simulink model "MedicalRoboticsProject"  (Simulink 8.5)
settings: Solver=ode4  StartTime=0.0  StopTime=20  FixedStep=0.01  RelTol=1e-3
model workspace (MAT data in the model file):
  Kx = 5
  Ky = 1.5
  Kz = 2
  x = 3
  y = 3
  z = 3
  K1 = 1
  K2 = 1
  K3 = 1
  K4 = 1
  K5 = 1
  K6 = 1
  Fx = 1
  Fy = 1
  Fz = 0.5
  F1 = 0
  F2 = -0.5
  F3 = 0
  xg = 4
  yg = 4
  zg : num (value not decoded)
values from neighbouring files (symbols this model uses):
  z = T(1:3,1:3)*z0    [DH.m]
settings Model: Creator=ahmad  LastModifiedBy=ahmad
settings DataIOCC: SignalLoggingSaveFormat=Dataset
settings OptimizationCC: ExpressionDepthLimit=128
settings DebuggingCC: UnderspecifiedInitializationDetection=Simplified  MergeDetectMultiDrivingBlocksExec=error  FcnCallInpInsideContextMsg=EnableAllAsError  StateNameClashWarn=none
settings GRTTargetCC: CombineOutputUpdateFcns=on  GRTInterface=off

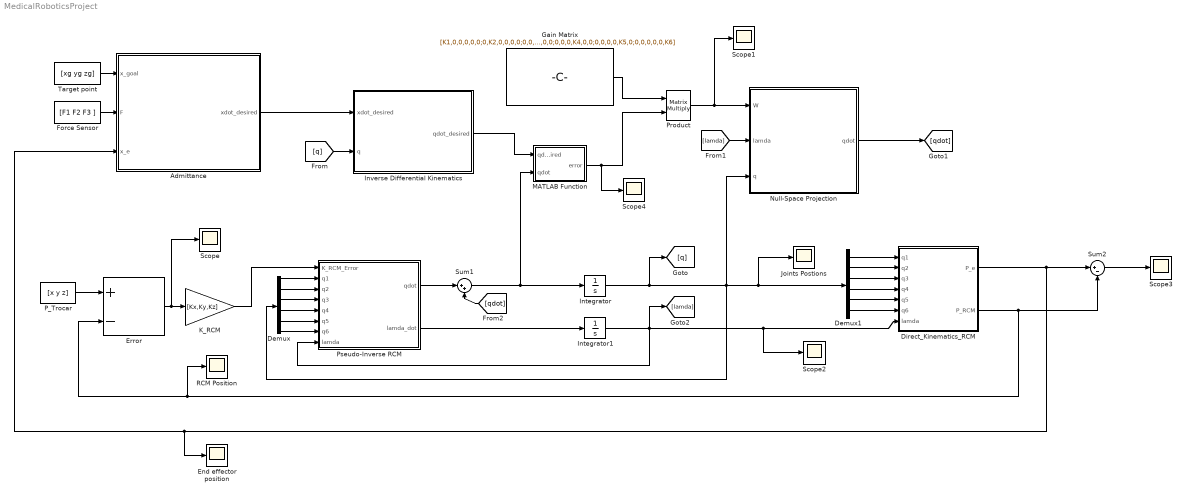
== system MedicalRoboticsProject ==
  Admittance : MATLAB Function  TreatAsAtomicUnit=on
  Demux : Demux  Outputs=6
  Demux1 : Demux  Outputs=6
  Direct_Kinematics_RCM : MATLAB Function  TreatAsAtomicUnit=on
  End effector position : Scope
      settings: YMin=-5e-12  YMax=2.5e-11  SaveName=ScopeData3
  Error : Sum  Inputs=+-
  Force Sensor : Constant  Value=[F1 F2 F3 ]
  Gain Matrix : Constant  Value=[K1,0,0,0,0,0;0,K2,0,0,0,0;0,0,K3,0,0,0;0,0,0,K4,0,0;0,0,0,0,K5,0;0,0,0,0,0,K6]  VectorParams1D=off
  Integrator : Integrator  InitialCondition=[1 1 1 pi/4 pi/4 1]
  Integrator1 : Integrator  InitialCondition=1  LimitOutput=on  UpperSaturationLimit=1  LowerSaturationLimit=0
  "Inverse Differential Kinematics " : MATLAB Function  TreatAsAtomicUnit=on
  Joints Postions : Scope
      settings: SaveName=ScopeData2
  K_RCM : Gain  Gain=[Kx,Ky,Kz]
  MATLAB Function : MATLAB Function  TreatAsAtomicUnit=on
  Null-Space Projection : MATLAB Function  TreatAsAtomicUnit=on
  P_Trocar : Constant  Value=[x y z]
  Product : Product  Multiplication=Matrix(*)
  "Pseudo-Inverse RCM " : MATLAB Function  TreatAsAtomicUnit=on
  RCM Position : Scope
      settings: YMin=-5e-12  YMax=2.5e-11  SaveName=ScopeData5
  Scope{,1..4} (5 alike) : Scope
      Scope settings: YMin=-5e-12  YMax=2.5e-11
      Scope2 settings: SaveName=ScopeData4
      Scope3 settings: SaveName=ScopeData6
      Scope4 settings: SaveName=ScopeData7
  Sum1 : Sum  Inputs=|++
  Sum2 : Sum  Inputs=|+-
  Target point : Constant  Value=[xg yg zg]
  wires:
  Demux/1 -> "Pseudo-Inverse RCM "/2(q1)
  Demux/2 -> "Pseudo-Inverse RCM "/3(q2)
  Demux/3 -> "Pseudo-Inverse RCM "/4(q3)
  Demux/4 -> "Pseudo-Inverse RCM "/5(q4)
  Demux/5 -> "Pseudo-Inverse RCM "/6(q5)
  Demux/6 -> "Pseudo-Inverse RCM "/7(q6)
  "Pseudo-Inverse RCM "/2(lamda_dot) -> Integrator1/1
  Integrator1/1 -> Scope2/1, Direct_Kinematics_RCM/7(lamda), [lamda], "Pseudo-Inverse RCM "/8(lamda)
  Integrator/1 -> [q], Null-Space Projection/3(q), Demux/1, Joints Postions/1, Demux1/1
  Demux1/1 -> Direct_Kinematics_RCM/1(q1)
  Demux1/2 -> Direct_Kinematics_RCM/2(q2)
  Demux1/3 -> Direct_Kinematics_RCM/3(q3)
  Demux1/4 -> Direct_Kinematics_RCM/4(q4)
  Demux1/5 -> Direct_Kinematics_RCM/5(q5)
  Demux1/6 -> Direct_Kinematics_RCM/6(q6)
  P_Trocar/1 -> Error/1
  Direct_Kinematics_RCM/2(P_RCM) -> RCM Position/1, Error/2, Sum2/2
  Error/1 -> Scope/1, K_RCM/1
  Target point/1 -> Admittance/1(x_goal)
  Force Sensor/1 -> Admittance/2(F)
  Admittance/1(xdot_desired) -> "Inverse Differential Kinematics "/1(xdot_desired)
  "Inverse Differential Kinematics "/1(qdot_desired) -> MATLAB Function/1(qdot_desired)
  "Pseudo-Inverse RCM "/1(qdot) -> Sum1/1
  [q] -> "Inverse Differential Kinematics "/2(q)
  [lamda] -> Null-Space Projection/2(lamda)
  Gain Matrix/1 -> Product/1
  Product/1 -> Null-Space Projection/1(W), Scope1/1
  Null-Space Projection/1(qdot) -> [qdot]
  K_RCM/1 -> "Pseudo-Inverse RCM "/1(K_RCM_Error)
  Sum1/1 -> Integrator/1, MATLAB Function/2(qdot)
  MATLAB Function/1(error) -> Scope4/1, Product/2
  Direct_Kinematics_RCM/1(P_e) -> Sum2/1, Admittance/3(x_e), End effector position/1
  [qdot] -> Sum1/2
  Sum2/1 -> Scope3/1

== matlab function Direct_Kinematics_RCM ==
  data: P_e output double; q1 input double; P_RCM output double; q2 input double; q3 input double; q4 input double; q5 input double; q6 input double; lamda input double
function [P_e, P_RCM]= fcn(q1, q2, q3, q4, q5, q6, lamda)
%#codegen
%p5 = [q2 + 5*sin(q4); q3 - (5*cos(q4)*(2^(1/2) + 2)^(1/2))/2 - 5*(2 - 2^(1/2))^(1/2); q1 + 5*(2^(1/2) + 2)^(1/2) - (5*cos(q4)*(2 - 2^(1/2))^(1/2))/2];
%p6 = [q2 + 5*sin(q4) - q6*cos(q4)*sin(q5); q3 - q6*((cos(q5)*(2 - 2^(1/2))^(1/2))/2 + (sin(q4)*sin(q5)*(2^(1/2) + 2)^(1/2))/2) - (5*cos(q4)*(2^(1/2) + 2)^(1/2))/2 - 5*(2 - 2^(1/2))^(1/2); q1 + 5*(2^(1/2) + 2)^(1/2) + q6*((cos(q5)*(2^(1/2) + 2)^(1/2))/2 - (sin(q4)*sin(q5)*(2 - 2^(1/2))^(1/2))/2) - (5*cos(q4)*(2 - 2^(1/2))^(1/2))/2];

p5 = [q2 + 5*cos(q4)*cos(q5)
      q3 - 5*(2 - 2^(1/2))^(1/2) - (5*sin(q5)*(2 - 2^(1/2))^(1/2))/2 + (5*cos(q5)*sin(q4)*(2^(1/2) + 2)^(1/2))/2
      q1 + 5*(2^(1/2) + 2)^(1/2) + (5*sin(q5)*(2^(1/2) + 2)^(1/2))/2 + (5*cos(q5)*sin(q4)*(2 - 2^(1/2))^(1/2))/2];
 

p6 =  [q2 + 5*cos(q4)*cos(q5) - q6*cos(q4)*sin(q5)
       q3 - q6*((cos(q5)*(2 - 2^(1/2))^(1/2))/2 + (sin(q4)*sin(q5)*(2^(1/2) + 2)^(1/2))/2) - 5*(2 - 2^(1/2))^(1/2) - (5*sin(q5)*(2 - 2^(1/2))^(1/2))/2 + (5*cos(q5)*sin(q4)*(2^(1/2) + 2)^(1/2))/2
       q1 + 5*(2^(1/2) + 2)^(1/2) + q6*((cos(q5)*(2^(1/2) + 2)^(1/2))/2 - (sin(q4)*sin(q5)*(2 - 2^(1/2))^(1/2))/2) + (5*sin(q5)*(2^(1/2) + 2)^(1/2))/2 + (5*cos(q5)*sin(q4)*(2 - 2^(1/2))^(1/2))/2];
 
P_RCM = p5 + lamda*(p6-p5);
P_e = p6;

== matlab function Pseudo-Inverse RCM  ==
  data: K_RCM_Error input double; q1 input double; q2 input double; q3 input double; q4 input double; qdot output double; q5 input double; q6 input double; lamda input double; lamda_dot output double
function [qdot,lamda_dot] = fcn(K_RCM_Error, q1, q2, q3, q4, q5, q6, lamda)
%#codegen
%coder.extrinsic('simplify'); 

% Jl1 = [0;0;1];
% Jl2 = [1;0;0];
% Jl3 = [0;1;0];
% Jl4 = [5*cos(q4) + q6*sin(q4)*sin(q5); ((5*sin(q4) - q6*cos(q4)*sin(q5))*(2^(1/2) + 2)^(1/2))/2; ((5*sin(q4) - q6*cos(q4)*sin(q5))*(2 - 2^(1/2))^(1/2))/2];

% Jl4 = simplify(Jl4);
% Jl5 = [-q6*cos(q4)*cos(q5); q6*((sin(q5)*(2 - 2^(1/2))^(1/2))/2 - (cos(q5)*sin(q4)*(2^(1/2) + 2)^(1/2))/2); -q6*((sin(q5)*(2^(1/2) + 2)^(1/2))/2 + (cos(q5)*sin(q4)*(2 - 2^(1/2))^(1/2))/2)];
% Jl5 = simplify(Jl5);
% Jl6 = [-cos(q4)*sin(q5);-(cos(q5)*(2 - 2^(1/2))^(1/2))/2 - (sin(q4)*sin(q5)*(2^(1/2) + 2)^(1/2))/2; (cos(q5)*(2^(1/2) + 2)^(1/2))/2 - (sin(q4)*sin(q5)*(2 - 2^(1/2))^(1/2))/2];
% Jl6 =  simplify(Jl6);


%J_5 = [0,1,0,5*cos(q4) + q6*sin(q4)*sin(q5),-q6*cos(q4)*cos(q5),0; 0,0,1,((5*sin(q4) - q6*cos(q4)*sin(q5))*(2^(1/2) + 2)^(1/2))/2,q6*((sin(q5)*(2 - 2^(1/2))^(1/2))/2 - (cos(q5)*sin(q4)*(2^(1/2) + 2)^(1/2))/2),0; 1,0,0,((5*sin(q4) - q6*cos(q4)*sin(q5))*(2 - 2^(1/2))^(1/2))/2,-q6*((sin(q5)*(2^(1/2) + 2)^(1/2))/2 + (cos(q5)*sin(q4)*(2 - 2^(1/2))^(1/2))/2),0];
% J_5 = [Jl1,Jl2,Jl3,Jl4,Jl5,0;0;0];
%J_6 = [Jl1,Jl2,Jl3,Jl4,Jl5,Jl6];
%J_6 = [0,1,0,5*cos(q4) + q6*sin(q4)*sin(q5),-q6*cos(q4)*cos(q5),-cos(q4)*sin(q5); 0,0,1,((5*sin(q4) - q6*cos(q4)*sin(q5))*(2^(1/2) + 2)^(1/2))/2,q6*((sin(q5)*(2 - 2^(1/2))^(1/2))/2 - (cos(q5)*sin(q4)*(2^(1/2) + 2)^(1/2))/2),-(cos(q5)*(2 - 2^(1/2))^(1/2))/2 - (sin(q4)*sin(q5)*(2^(1/2) + 2)^(1/2))/2; 1,0,0,((5*sin(q4) - q6*cos(q4)*sin(q5))*(2 - 2^(1/2))^(1/2))/2,-q6*((sin(q5)*(2^(1/2) + 2)^(1/2))/2 + (cos(q5)*sin(q4)*(2 - 2^(1/2))^(1/2))/2),(cos(q5)*(2^(1/2) + 2)^(1/2))/2 - (sin(q4)*sin(q5)*(2 - 2^(1/2))^(1/2))/2];

J_5 = [0, 1, 0, -sin(q4)*(5*cos(q5) - q6*sin(q5)), -cos(q4)*(5*sin(q5) + q6*cos(q5)), 0
       0, 0, 1, (cos(q4)*(5*cos(q5) - q6*sin(q5))*(2^(1/2) + 2)^(1/2))/2, q6*((sin(q5)*(2 - 2^(1/2))^(1/2))/2 - (cos(q5)*sin(q4)*(2^(1/2) + 2)^(1/2))/2) - (5*cos(q5)*(2 - 2^(1/2))^(1/2))/2 - (5*sin(q4)*sin(q5)*(2^(1/2) + 2)^(1/2))/2, 0
       1, 0, 0, (cos(q4)*(5*cos(q5) - q6*sin(q5))*(2 - 2^(1/2))^(1/2))/2, (5*cos(q5)*(2^(1/2) + 2)^(1/2))/2 - q6*((sin(q5)*(2^(1/2) + 2)^(1/2))/2 + (cos(q5)*sin(q4)*(2 - 2^(1/2))^(1/2))/2) - (5*sin(q4)*sin(q5)*(2 - 2^(1/2))^(1/2))/2, 0];

J_6 = [0, 1, 0, -sin(q4)*(5*cos(q5) - q6*sin(q5)), -cos(q4)*(5*sin(q5) + q6*cos(q5)), -cos(q4)*sin(q5)
       0, 0, 1, (cos(q4)*(5*cos(q5) - q6*sin(q5))*(2^(1/2) + 2)^(1/2))/2, q6*((sin(q5)*(2 - 2^(1/2))^(1/2))/2 - (cos(q5)*sin(q4)*(2^(1/2) + 2)^(1/2))/2) - (5*cos(q5)*(2 - 2^(1/2))^(1/2))/2 - (5*sin(q4)*sin(q5)*(2^(1/2) + 2)^(1/2))/2, - (cos(q5)*(2 - 2^(1/2))^(1/2))/2 - (sin(q4)*sin(q5)*(2^(1/2) + 2)^(1/2))/2
       1, 0, 0, (cos(q4)*(5*cos(q5) - q6*sin(q5))*(2 - 2^(1/2))^(1/2))/2, (5*cos(q5)*(2^(1/2) + 2)^(1/2))/2 - q6*((sin(q5)*(2^(1/2) + 2)^(1/2))/2 + (cos(q5)*sin(q4)*(2 - 2^(1/2))^(1/2))/2) - (5*sin(q4)*sin(q5)*(2 - 2^(1/2))^(1/2))/2,   (cos(q5)*(2^(1/2) + 2)^(1/2))/2 - (sin(q4)*sin(q5)*(2 - 2^(1/2))^(1/2))/2];

temp1 = (J_5 + lamda*(J_6-J_5));
qdot = pinv(temp1)* K_RCM_Error;

p5 = [q2 + 5*sin(q4); q3 - (5*cos(q4)*(2^(1/2) + 2)^(1/2))/2 - 5*(2 - 2^(1/2))^(1/2); q1 + 5*(2^(1/2) + 2)^(1/2) - (5*cos(q4)*(2 - 2^(1/2))^(1/2))/2];
p6 = [q2 + 5*sin(q4) - q6*cos(q4)*sin(q5); q3 - q6*((cos(q5)*(2 - 2^(1/2))^(1/2))/2 + (sin(q4)*sin(q5)*(2^(1/2) + 2)^(1/2))/2) - (5*cos(q4)*(2^(1/2) + 2)^(1/2))/2 - 5*(2 - 2^(1/2))^(1/2); q1 + 5*(2^(1/2) + 2)^(1/2) + q6*((cos(q5)*(2^(1/2) + 2)^(1/2))/2 - (sin(q4)*sin(q5)*(2 - 2^(1/2))^(1/2))/2) - (5*cos(q4)*(2 - 2^(1/2))^(1/2))/2];
temp2 = p6-p5;
lamda_dot = 1/(temp2)* K_RCM_Error;

== matlab function Admittance ==
  data: x_goal input double; xdot_desired output double; F input double; x_e input double
function xdot_desired = fcn(x_goal, F, x_e)
%#codegen
delta = x_goal - x_e;
F_delta = (delta.'* F * delta)/(norm(delta,2));
xdot_desired = 0.5*F_delta; %hard virtual-fixtures, where Ct = 0, and C = 0.5 for scaling the surgeon speed of insertion

== matlab function Inverse Differential Kinematics  ==
  data: xdot_desired input double; qdot_desired output double; q input double
function qdot_desired = fcn(xdot_desired, q)
%#codegen
qdot_desired = zeros(6,1);
%J_6 = [0,1,0,5*cos(q(4)) + q(6)*sin(q(4))*sin(q(5)),-q(6)*cos(q(4))*cos(q(5)),-cos(q(4))*sin(q(5)); 0,0,1,((5*sin(q(4)) - q(6)*cos(q(4))*sin(q(5)))*(2^(1/2) + 2)^(1/2))/2,q(6)*((sin(q(5))*(2 - 2^(1/2))^(1/2))/2 - (cos(q(5))*sin(q(4))*(2^(1/2) + 2)^(1/2))/2),-(cos(q(5))*(2 - 2^(1/2))^(1/2))/2 - (sin(q(4))*sin(q(5))*(2^(1/2) + 2)^(1/2))/2; 1,0,0,((5*sin(q(4)) - q(6)*cos(q(4))*sin(q(5)))*(2 - 2^(1/2))^(1/2))/2,-q(6)*((sin(q(5))*(2^(1/2) + 2)^(1/2))/2 + (cos(q(5))*sin(q(4))*(2 - 2^(1/2))^(1/2))/2),(cos(q(5))*(2^(1/2) + 2)^(1/2))/2 - (sin(q(4))*sin(q(5))*(2 - 2^(1/2))^(1/2))/2];
J_6 = [0, 1, 0, -sin(q(4))*(5*cos(q(5)) - q(6)*sin(q(5))), -cos(q(4))*(5*sin(q(5)) + q(6)*cos(q(5))), -cos(q(4))*sin(q(5))
       0, 0, 1, (cos(q(4))*(5*cos(q(5)) - q(6)*sin(q(5)))*(2^(1/2) + 2)^(1/2))/2, q(6)*((sin(q(5))*(2 - 2^(1/2))^(1/2))/2 - (cos(q(5))*sin(q(4))*(2^(1/2) + 2)^(1/2))/2) - (5*cos(q(5))*(2 - 2^(1/2))^(1/2))/2 - (5*sin(q(4))*sin(q(5))*(2^(1/2) + 2)^(1/2))/2, - (cos(q(5))*(2 - 2^(1/2))^(1/2))/2 - (sin(q(4))*sin(q(5))*(2^(1/2) + 2)^(1/2))/2
       1, 0, 0, (cos(q(4))*(5*cos(q(5)) - q(6)*sin(q(5)))*(2 - 2^(1/2))^(1/2))/2, (5*cos(q(5))*(2^(1/2) + 2)^(1/2))/2 - q(6)*((sin(q(5))*(2^(1/2) + 2)^(1/2))/2 + (cos(q(5))*sin(q(4))*(2 - 2^(1/2))^(1/2))/2) - (5*sin(q(4))*sin(q(5))*(2 - 2^(1/2))^(1/2))/2,   (cos(q(5))*(2^(1/2) + 2)^(1/2))/2 - (sin(q(4))*sin(q(5))*(2 - 2^(1/2))^(1/2))/2];
pseudo = pinv(J_6);
qdot_desired = pseudo*xdot_desired;

== matlab function Null-Space Projection ==
  data: W input double; qdot output double; lamda input double; q input double
function qdot = fcn(W, lamda, q)
%#codegen
qdot = zeros(6,1);
%J_5 = [0,1,0,5*cos(q(4)) + q(6)*sin(q(4))*sin(q(5)),-q(6)*cos(q(4))*cos(q(5)),0; 0,0,1,((5*sin(q(4)) - q(6)*cos(q(4))*sin(q(5)))*(2^(1/2) + 2)^(1/2))/2,q(6)*((sin(q(5))*(2 - 2^(1/2))^(1/2))/2 - (cos(q(5))*sin(q(4))*(2^(1/2) + 2)^(1/2))/2),0; 1,0,0,((5*sin(q(4)) - q(6)*cos(q(4))*sin(q(5)))*(2 - 2^(1/2))^(1/2))/2,-q(6)*((sin(q(5))*(2^(1/2) + 2)^(1/2))/2 + (cos(q(5))*sin(q(4))*(2 - 2^(1/2))^(1/2))/2),0];
%J_6 = [0,1,0,5*cos(q(4)) + q(6)*sin(q(4))*sin(q(5)),-q(6)*cos(q(4))*cos(q(5)),-cos(q(4))*sin(q(5)); 0,0,1,((5*sin(q(4)) - q(6)*cos(q(4))*sin(q(5)))*(2^(1/2) + 2)^(1/2))/2,q(6)*((sin(q(5))*(2 - 2^(1/2))^(1/2))/2 - (cos(q(5))*sin(q(4))*(2^(1/2) + 2)^(1/2))/2),-(cos(q(5))*(2 - 2^(1/2))^(1/2))/2 - (sin(q(4))*sin(q(5))*(2^(1/2) + 2)^(1/2))/2; 1,0,0,((5*sin(q(4)) - q(6)*cos(q(4))*sin(q(5)))*(2 - 2^(1/2))^(1/2))/2,-q(6)*((sin(q(5))*(2^(1/2) + 2)^(1/2))/2 + (cos(q(5))*sin(q(4))*(2 - 2^(1/2))^(1/2))/2),(cos(q(5))*(2^(1/2) + 2)^(1/2))/2 - (sin(q(4))*sin(q(5))*(2 - 2^(1/2))^(1/2))/2];

J_5 = [0, 1, 0, -sin(q(4))*(5*cos(q(5)) - q(6)*sin(q(5))), -cos(q(4))*(5*sin(q(5)) + q(6)*cos(q(5))), 0
       0, 0, 1, (cos(q(4))*(5*cos(q(5)) - q(6)*sin(q(5)))*(2^(1/2) + 2)^(1/2))/2, q(6)*((sin(q(5))*(2 - 2^(1/2))^(1/2))/2 - (cos(q(5))*sin(q(4))*(2^(1/2) + 2)^(1/2))/2) - (5*cos(q(5))*(2 - 2^(1/2))^(1/2))/2 - (5*sin(q(4))*sin(q(5))*(2^(1/2) + 2)^(1/2))/2, 0
       1, 0, 0, (cos(q(4))*(5*cos(q(5)) - q(6)*sin(q(5)))*(2 - 2^(1/2))^(1/2))/2, (5*cos(q(5))*(2^(1/2) + 2)^(1/2))/2 - q(6)*((sin(q(5))*(2^(1/2) + 2)^(1/2))/2 + (cos(q(5))*sin(q(4))*(2 - 2^(1/2))^(1/2))/2) - (5*sin(q(4))*sin(q(5))*(2 - 2^(1/2))^(1/2))/2, 0];


J_6 = [0, 1, 0, -sin(q(4))*(5*cos(q(5)) - q(6)*sin(q(5))), -cos(q(4))*(5*sin(q(5)) + q(6)*cos(q(5))), -cos(q(4))*sin(q(5))
       0, 0, 1, (cos(q(4))*(5*cos(q(5)) - q(6)*sin(q(5)))*(2^(1/2) + 2)^(1/2))/2, q(6)*((sin(q(5))*(2 - 2^(1/2))^(1/2))/2 - (cos(q(5))*sin(q(4))*(2^(1/2) + 2)^(1/2))/2) - (5*cos(q(5))*(2 - 2^(1/2))^(1/2))/2 - (5*sin(q(4))*sin(q(5))*(2^(1/2) + 2)^(1/2))/2, - (cos(q(5))*(2 - 2^(1/2))^(1/2))/2 - (sin(q(4))*sin(q(5))*(2^(1/2) + 2)^(1/2))/2
       1, 0, 0, (cos(q(4))*(5*cos(q(5)) - q(6)*sin(q(5)))*(2 - 2^(1/2))^(1/2))/2, (5*cos(q(5))*(2^(1/2) + 2)^(1/2))/2 - q(6)*((sin(q(5))*(2^(1/2) + 2)^(1/2))/2 + (cos(q(5))*sin(q(4))*(2 - 2^(1/2))^(1/2))/2) - (5*sin(q(4))*sin(q(5))*(2 - 2^(1/2))^(1/2))/2,   (cos(q(5))*(2^(1/2) + 2)^(1/2))/2 - (sin(q(4))*sin(q(5))*(2 - 2^(1/2))^(1/2))/2];

Jrcm = (J_5 + lamda*(J_6-J_5));
pseudo = pinv(Jrcm);
qdot = (eye(6)-(pseudo*Jrcm))*W;

== matlab function MATLAB Function ==
  data: qdot_desired input double; error output double; qdot input double
function error = fcn(qdot_desired, qdot)
%#codegen
error = qdot_desired - qdot;
